simulink model "Main_2015a_ABS"  (R2015a)
settings: Solver=ode45  SolverMode=SingleTasking  StartTime=0.0  StopTime=20  MaxStep=.01  RelTol=1e-3  AbsTol=1e-6
PreLoadFcn:
  | % Load initialization data
  | 
  | sldemo_absdata;
values from neighbouring files (symbols this model uses):
  ABS_FLAG = 1    [matlab.mat]
  g = 9.8    [matlab.mat]
  I = 1.04    [matlab.mat]
  Kf = 1    [matlab.mat]
  m = 350    [matlab.mat]
  mu = [0 0.4 0.8 0.97 1 0.98 0.96 0.94 0.92 0.9 0.88 0.855 ... (21 elements, 1x21)]    [matlab.mat]
  PBmax = 1500    [matlab.mat]
  Rr = 0.356    [matlab.mat]
  slip = [0 0.05 0.1 0.15 0.2 0.25 0.3 0.35 0.4 0.45 0.5 0.55 ... (21 elements, 1x21)]    [matlab.mat]
  TB = 0.01    [matlab.mat]
  v0 = 22    [matlab.mat]
libraries: simulink_extras x4
CloseFcn:
  | % Close the plots that are still open
  | h = findobj(0, 'Name', 'ABS Speeds');
  | if ~isempty(h),
  |   close(h);
  | end;
  | 
  | h = findobj(0, 'Name', 'ABS Slip');
  | if ~isempty(h),
  |   close(h);
  | end;
  | 
  | % Clear initial conditions data to avoid cluttering the workspace
  | 
  | clear g v0 Rr Kf m PBmax TB I slip mu ctrl h;
Description:
  | Modeling an Anti-Lock Braking System (ABS)
  | 
  | *Summary*
  | 
  | This example describes a simple model for an Anti-Lock Braking System
  | (ABS). The model simulates the dynamic behavior of a vehicle
  | under hard braking conditions. The model represents a single wheel, which
  | may be replicated a number of times to create a model for a multi-wheel
  | vehicle.
  | 
  | This model uses the signal logging feature in Simulink(R). You log signals to the
  | MATLAB(R) workspace where you can analyze and view them. You can view
  | the code in sldemo_absbrakeplots.m to see how this is done.
  | 
  | In this model, the wheel speed is calculated in a separate component
  | named sldemo_wheelspeed_absbrake.
  | This component is then referenced using a Model block.  Note that both the
  | top model and the referenced model use a variable step solver, so Simulink
  | will track zero-crossings in the referenced model.
settings Model: FPTRunName=Active  CovSFcnEnable=off  ExtModeTrigMode=oneshot  ExtModeArmWhenConnect=off  ExtModeAutoUpdateStatusClock=off  Creator=The MathWorks, Inc.  LastModifiedBy=kankan
settings DataIOCC: LimitDataPoints=off  SaveOutput=off  SaveTime=off  TimeSaveName=time  SignalLoggingName=sldemo_absbrake_output
settings OptimizationCC: InlineParams=on  InlineInvariantSignals=on  ExpressionDepthLimit=2147483647  InitFltsAndDblsToZero=on  BufferReusableBoundary=off
settings DebuggingCC: SaveWithParameterizedLinksMsg=none  MultiTaskDSMMsg=warning  SigSpecEnsureSampleTimeMsg=none  IntegerOverflowMsg=none  FcnCallInpInsideContextMsg=EnableAllAsWarning  BusObjectLabelMismatch=none  StateNameClashWarn=warning  IntegerSaturationMsg=none
settings HardwareCC: TargetBitPerPointer=64  TargetLongLongMode=on  TargetIntDivRoundTo=Zero  TargetEndianess=LittleEndian  TargetWordSize=64  TargetHWDeviceType=MATLAB Host
settings ModelReferenceCC: UpdateModelReferenceTargets=IfOutOfDate

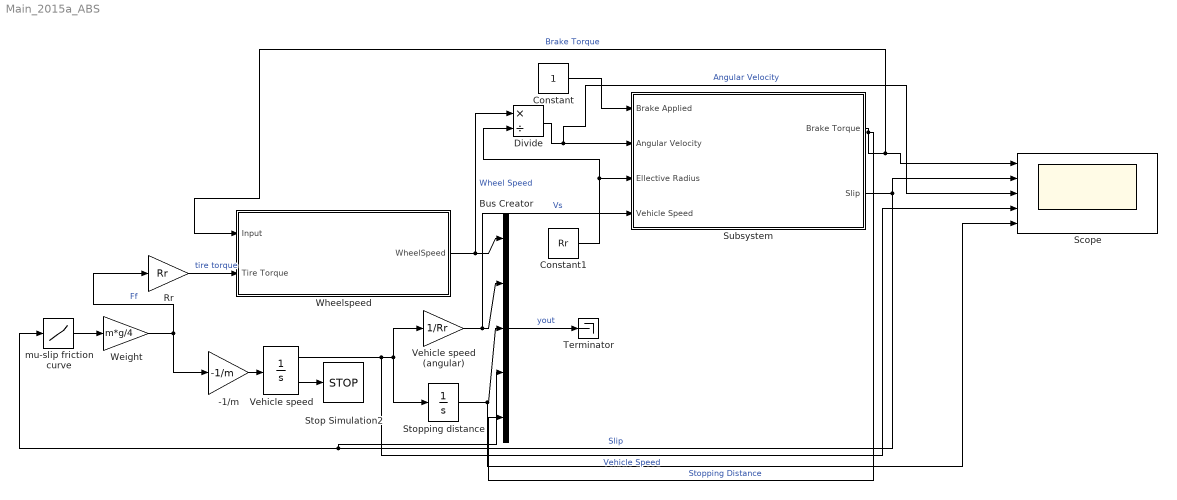
== system Main_2015a_ABS ==
  -1/m : Gain  Gain=-1/m  SaturateOnIntegerOverflow=on  OutDataTypeStr=Inherit: Same as input  ParamDataTypeStr=Inherit: Same as input
  Bus Creator : BusCreator  Inputs=5
  Constant : Constant
  Constant1 : Constant  Value=Rr
  Divide : Product  Inputs=*/
  Rr : Gain  Gain=Rr  SaturateOnIntegerOverflow=on  OutDataTypeStr=Inherit: Same as input  ParamDataTypeStr=Inherit: Same as input
  Scope : Scope  NumInputPorts=5
      settings: TimeRange=auto  MaxDataPoints=5000  SaveToWorkspace=off  SaveName=ScopeData  YMin=-2.5~-0.125~-21.69865~-2.73894~-16.73211  YMax=2.5~1.125~195.28784~24.74877~150.58895  SampleTime=-1
  Stop Simulation2 : Stop
  Stopping distance : Integrator  UpperSaturationLimit=1000  LowerSaturationLimit=0
  Subsystem : Subsystem
  Terminator : Terminator
  Vehicle speed : Integrator  InitialCondition=v0  LimitOutput=on  UpperSaturationLimit=1000  LowerSaturationLimit=0  ShowSaturationPort=on
  Vehicle speed (angular) : Gain  Gain=1/Rr  SaturateOnIntegerOverflow=on  OutDataTypeStr=Inherit: Same as input  ParamDataTypeStr=Inherit: Same as input
  Weight : Gain  Gain=m*g/4  SaturateOnIntegerOverflow=on  OutDataTypeStr=Inherit: Same as input  ParamDataTypeStr=Inherit: Same as input
  "Wheelspeed " : Subsystem
  mu-slip friction curve : Lookup_n-D  NumberOfTableDimensions=1  BreakpointsForDimension1=slip  Table=mu  SaturateOnIntegerOverflow=on  InputSameDT=on
  wires:
  Vehicle speed (angular)/1 -> Bus Creator/2, Subsystem/4(Vehicle Speed)  "Vs"
  Stopping distance/1 -> Scope/5, Bus Creator/3  "Stopping Distance"
  -1/m/1 -> Vehicle speed/1
  Vehicle speed/2 -> Stop Simulation2/1
  Vehicle speed/1 -> Scope/4, Stopping distance/1, Vehicle speed (angular)/1  "Vehicle Speed"
  mu-slip friction curve/1 -> Weight/1
  Weight/1 -> -1/m/1, Rr/1  "Ff"
  "Wheelspeed "/1(WheelSpeed) -> Divide/1, Bus Creator/1  "Wheel Speed"
  Rr/1 -> "Wheelspeed "/2(Tire Torque)  "tire torque"
  Constant/1 -> Subsystem/1(Brake Applied)
  Divide/1 -> Scope/3, Subsystem/2(Angular Velocity)  "Angular Velocity"
  Constant1/1 -> Subsystem/3(Ellective Radius), Divide/2
  Subsystem/1(Brake Torque) -> Bus Creator/5, "Wheelspeed "/1(Input), Scope/1  "Brake Torque"
  Subsystem/2(Slip) -> Scope/2, Bus Creator/4, mu-slip friction curve/1  "Slip"
  Bus Creator/1 -> Terminator/1  "yout"

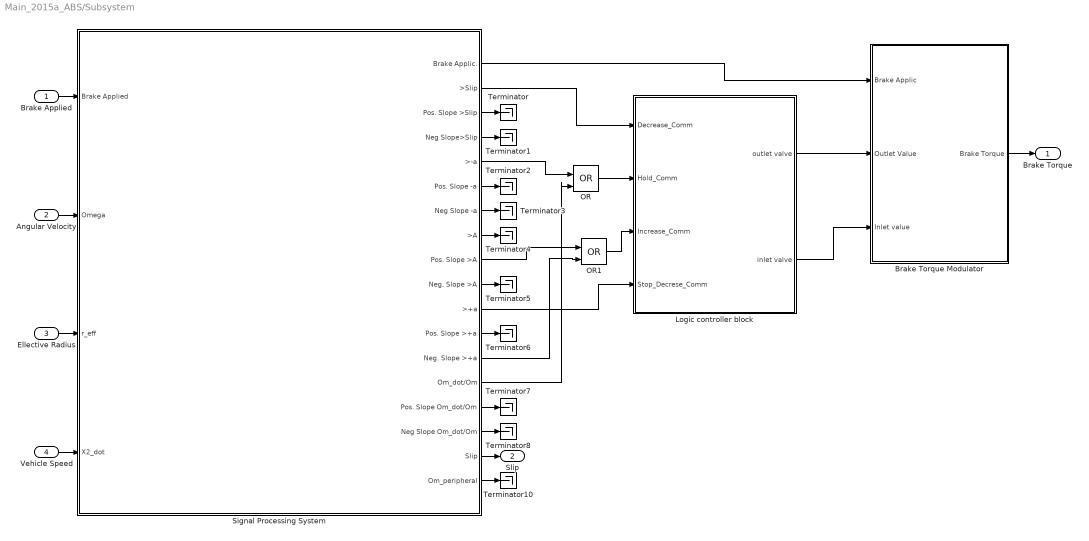
== system Main_2015a_ABS/Subsystem ==
  Brake Applied : Inport
  Angular Velocity : Inport  Port=2
  Ellective Radius : Inport  Port=3
  Vehicle Speed : Inport  Port=4
  "Brake Torque Modulator " : Subsystem
  Logic controller block : Subsystem
  OR : Logic  Operator=OR  IconShape=distinctive  AllPortsSameDT=off  OutDataTypeStr=boolean
  OR1 : Logic  Operator=OR  IconShape=distinctive  AllPortsSameDT=off  OutDataTypeStr=boolean
  Signal Processing System : Subsystem
  Terminator{,1..8,10} (10 alike) : Terminator
  Brake Torque : Outport
  Slip : Outport  Port=2
  wires:
  OR1/1 -> Logic controller block/3(Increase_Comm)
  Signal Processing System/8(>A) -> Terminator4/1
  Vehicle Speed/1 -> Signal Processing System/4(X2_dot)
  Signal Processing System/1(Brake Applic.) -> "Brake Torque Modulator "/1(Brake Applic)
  Signal Processing System/5(>-a) -> OR/1
  Brake Applied/1 -> Signal Processing System/1(Brake Applied)
  OR/1 -> Logic controller block/2(Hold_Comm)
  Signal Processing System/13(Neg. Slope >+a) -> OR1/2
  Signal Processing System/9(Pos. Slope >A) -> OR1/1
  Signal Processing System/6(Pos. Slope -a) -> Terminator2/1
  Signal Processing System/11(>+a) -> Logic controller block/4(Stop_Decrese_Comm)
  Signal Processing System/2(>Slip) -> Logic controller block/1(Decrease_Comm)
  Ellective Radius/1 -> Signal Processing System/3(r_eff)
  Logic controller block/1("outlet valve ") -> "Brake Torque Modulator "/2(Outlet Value)
  Logic controller block/2("inlet valve ") -> "Brake Torque Modulator "/3(Inlet value)
  Signal Processing System/4(Neg Slope>Slip) -> Terminator1/1
  Signal Processing System/14(Om_dot/Om) -> OR/2
  Signal Processing System/10(Neg. Slope >A) -> Terminator5/1
  Signal Processing System/12(Pos. Slope >+a) -> Terminator6/1
  Signal Processing System/15(Pos. Slope Om_dot/Om) -> Terminator7/1
  Signal Processing System/16(Neg Slope Om_dot/Om) -> Terminator8/1
  "Brake Torque Modulator "/1(Brake Torque) -> Brake Torque/1
  Signal Processing System/18("Om_peripheral ") -> Terminator10/1
  Signal Processing System/17(Slip) -> Slip/1
  Signal Processing System/7(Neg Slope -a) -> Terminator3/1
  Signal Processing System/3(Pos. Slope >Slip) -> Terminator/1
  Angular Velocity/1 -> Signal Processing System/2(Omega)

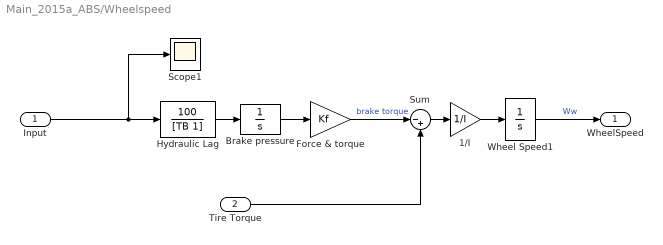
== system Main_2015a_ABS/Wheelspeed  ==
  Input : Inport  SampleTime=0
  Tire Torque : Inport  Port=2
  1/I : Gain  Gain=1/I  SaturateOnIntegerOverflow=on  OutDataTypeStr=Inherit: Same as input  ParamDataTypeStr=Inherit: Same as input
  Brake pressure : Integrator  LimitOutput=on  UpperSaturationLimit=PBmax  LowerSaturationLimit=0
  Force & torque : Gain  Gain=Kf  SaturateOnIntegerOverflow=on  OutDataTypeStr=Inherit: Same as input  ParamDataTypeStr=Inherit: Same as input
  "Hydraulic Lag " : TransferFcn  Numerator=[100]  Denominator=[TB 1]
  Scope1 : Scope
      settings: TimeRange=auto  MaxDataPoints=5000  SaveToWorkspace=off  YMin=-1.25  YMax=1.25  SampleTime=-1
  Sum : Sum  Inputs=|-+  SaturateOnIntegerOverflow=on  InputSameDT=on  OutDataTypeStr=Inherit: Same as first input
  Wheel Speed1 : Integrator  InitialCondition=v0/Rr  LimitOutput=on  UpperSaturationLimit=1000  LowerSaturationLimit=0
  WheelSpeed : Outport
  wires:
  Tire Torque/1 -> Sum/2
  Sum/1 -> 1/I/1
  Force & torque/1 -> Sum/1  "brake torque"
  "Hydraulic Lag "/1 -> Brake pressure/1
  1/I/1 -> Wheel Speed1/1
  Wheel Speed1/1 -> WheelSpeed/1  "Ww"
  Input/1 -> Scope1/1, "Hydraulic Lag "/1
  Brake pressure/1 -> Force & torque/1

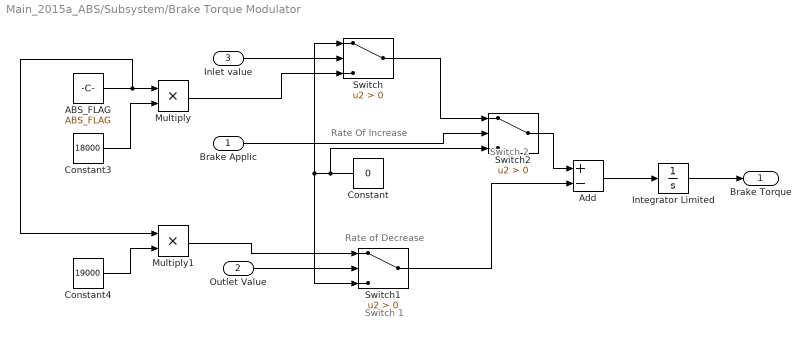
== system Main_2015a_ABS/Subsystem/Brake Torque Modulator  ==
  note: Switch 2
  note: Rate Of Increase
  note: Switch 1
  note: Rate of Decrease
  Brake Applic : Inport
  Outlet Value : Inport  Port=2
  Inlet value : Inport  Port=3
  ABS_FLAG : Constant  Value=ABS_FLAG
  Add : Sum  Inputs=+-
  Constant : Constant  Value=0
  Constant3 : Constant  Value=18000
  Constant4 : Constant  Value=19000
  Integrator Limited : Integrator  InitialCondition=1  LimitOutput=on  UpperSaturationLimit=2  LowerSaturationLimit=-2  ContinuousStateAttributes='RPM'
  Multiply : Product
  Multiply1 : Product
  Switch : Switch  Criteria=u2 > Threshold
  Switch1 : Switch  Criteria=u2 > Threshold
  Switch2 : Switch  Criteria=u2 > Threshold
  Brake Torque : Outport
  wires:
  Integrator Limited/1 -> Brake Torque/1
  Add/1 -> Integrator Limited/1
  Switch1/1 -> Add/2
  Switch2/1 -> Add/1
  Switch/1 -> Switch2/1
  Constant/1 -> Switch2/3, Switch/1, Switch1/3
  Brake Applic/1 -> Switch2/2
  Inlet value/1 -> Switch/2
  Outlet Value/1 -> Switch1/2
  ABS_FLAG/1 -> Multiply1/1, Multiply/1
  Constant3/1 -> Multiply/2
  Multiply/1 -> Switch/3
  Multiply1/1 -> Switch1/1
  Constant4/1 -> Multiply1/2

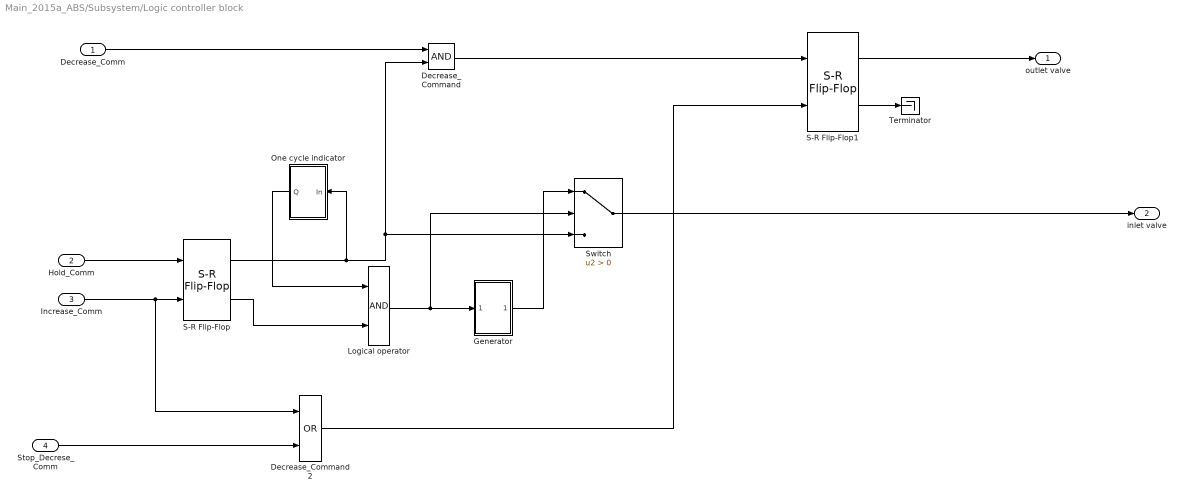
== system Main_2015a_ABS/Subsystem/Logic controller block ==
  Decrease_Comm : Inport
  Hold_Comm : Inport  Port=2
  Increase_Comm : Inport  Port=3
  Stop_Decrese_Comm : Inport  Port=4
  "Decrease_Command " : Logic  AllPortsSameDT=off  OutDataTypeStr=boolean
  Decrease_Command 2 : Logic  Operator=OR  AllPortsSameDT=off  OutDataTypeStr=boolean
  Generator : Subsystem
  "Logical operator " : Logic  AllPortsSameDT=off  OutDataTypeStr=boolean
  One cycle indicator : Subsystem
  S-R Flip-Flop : simulink_extras/Flip Flops/S-R Flip-Flop  initial_condition=0
  S-R Flip-Flop1 : simulink_extras/Flip Flops/S-R Flip-Flop  initial_condition=0
  Switch : Switch  Criteria=u2 > Threshold
  Terminator : Terminator
  "outlet valve " : Outport
  "inlet valve " : Outport  Port=2
  wires:
  Hold_Comm/1 -> S-R Flip-Flop/1
  Increase_Comm/1 -> Decrease_Command 2/1, S-R Flip-Flop/2
  Decrease_Comm/1 -> "Decrease_Command "/1
  S-R Flip-Flop/1 -> One cycle indicator/1("In "), Switch/3, "Decrease_Command "/2
  One cycle indicator/1(Q) -> "Logical operator "/1
  S-R Flip-Flop1/1 -> "outlet valve "/1
  "Decrease_Command "/1 -> S-R Flip-Flop1/1
  Switch/1 -> "inlet valve "/1
  "Logical operator "/1 -> Switch/2, Generator/1(In1)
  Stop_Decrese_Comm/1 -> Decrease_Command 2/2
  Decrease_Command 2/1 -> S-R Flip-Flop1/2
  Generator/1("out ") -> Switch/1
  S-R Flip-Flop1/2 -> Terminator/1
  S-R Flip-Flop/2 -> "Logical operator "/2

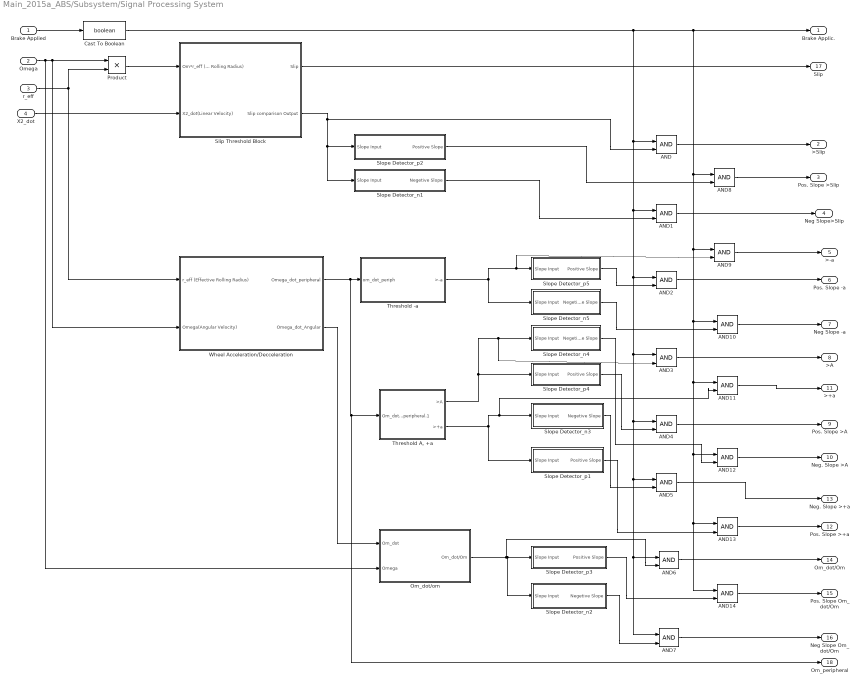
== system Main_2015a_ABS/Subsystem/Signal Processing System ==
  Brake Applied : Inport
  Omega : Inport  Port=2
  r_eff : Inport  Port=3
  X2_dot : Inport  Port=4
  AND{,1..14} (15 alike) : Logic  IconShape=distinctive  AllPortsSameDT=off  OutDataTypeStr=boolean
  Cast To Boolean : DataTypeConversion  OutDataTypeStr=boolean
  Om_dot/om : Subsystem
  Product : Product
  Slip Threshold Block : Subsystem
  Slope Detector_n1 : Subsystem
  Slope Detector_n2 : Subsystem
  Slope Detector_n3 : Subsystem
  Slope Detector_n4 : Subsystem
  Slope Detector_n5 : Subsystem
  Slope Detector_p1 : Subsystem
  Slope Detector_p2 : Subsystem
  Slope Detector_p3 : Subsystem
  Slope Detector_p4 : Subsystem
  Slope Detector_p5 : Subsystem
  Threshold -a : Subsystem
  "Threshold A, +a" : Subsystem
  Wheel Acceleration/Decceleration : Subsystem
  Brake Applic. : Outport
  >Slip : Outport  Port=2
  Pos. Slope >Slip : Outport  Port=3
  Neg Slope>Slip : Outport  Port=4
  >-a : Outport  Port=5
  Pos. Slope -a : Outport  Port=6
  Neg Slope -a : Outport  Port=7
  >A : Outport  Port=8
  Pos. Slope >A : Outport  Port=9
  Neg. Slope >A : Outport  Port=10
  >+a : Outport  Port=11
  Pos. Slope >+a : Outport  Port=12
  Neg. Slope >+a : Outport  Port=13
  Om_dot/Om : Outport  Port=14
  Pos. Slope Om_dot/Om : Outport  Port=15
  Neg Slope Om_dot/Om : Outport  Port=16
  Slip : Outport  Port=17
  "Om_peripheral " : Outport  Port=18
  wires:
  "Threshold A, +a"/2(>+a) -> AND11/2, Slope Detector_n3/1(Slope Input), Slope Detector_p1/1(Slope Input)
  Threshold -a/1(>-a) -> Slope Detector_n5/1(Slope Input), AND9/2, Slope Detector_p5/1(Slope Input)
  AND4/1 -> Pos. Slope >A/1
  AND/1 -> >Slip/1
  Product/1 -> Slip Threshold Block/1(Om*r_eff (Angular Velocity * Rolling Radius))
  Brake Applied/1 -> Cast To Boolean/1
  AND3/1 -> >A/1
  Cast To Boolean/1 -> AND/1, AND1/1, AND2/1, AND3/1, AND4/1, AND5/1, AND6/1, AND7/1, Brake Applic./1, AND8/1, AND9/1, AND10/1, AND12/1, AND13/1, AND14/1, AND11/1
  Slope Detector_n5/1(Negetive Slope) -> AND10/2
  Slip Threshold Block/2(Slip comparison Output) -> AND/2, Slope Detector_n1/1(Slope Input), Slope Detector_p2/1(Slope Input)
  r_eff/1 -> Wheel Acceleration/Decceleration/1(r_eff (Effective Rolling Radius)), Product/2
  "Threshold A, +a"/1(>A) -> AND3/2, Slope Detector_n4/1(Slope Input), Slope Detector_p4/1(Slope Input)
  Slope Detector_p2/1(Positive Slope) -> AND8/2
  AND6/1 -> Om_dot/Om/1
  Slope Detector_n2/1(Negetive Slope) -> AND7/2
  AND1/1 -> Neg Slope>Slip/1
  AND13/1 -> Pos. Slope >+a/1
  AND5/1 -> Neg. Slope >+a/1
  AND12/1 -> Neg. Slope >A/1
  AND14/1 -> Pos. Slope Om_dot/Om/1
  Om_dot/om/1(Om_dot/Om) -> AND6/2, Slope Detector_n2/1(Slope Input), Slope Detector_p3/1(Slope Input)
  Slope Detector_p5/1(Positive Slope) -> AND2/2
  AND9/1 -> >-a/1
  Omega/1 -> Om_dot/om/2(Omega), Wheel Acceleration/Decceleration/2(Omega(Angular Velocity)), Product/1
  Wheel Acceleration/Decceleration/2(Omega_dot_Angular) -> Om_dot/om/1(Om_dot)
  Slope Detector_p1/1(Positive Slope) -> AND13/2
  Slope Detector_p3/1(Positive Slope) -> AND14/2
  Slope Detector_n1/1(Negetive Slope) -> AND1/2
  AND2/1 -> Pos. Slope -a/1
  AND10/1 -> Neg Slope -a/1
  Wheel Acceleration/Decceleration/1(Omega_dot_peripheral) -> Threshold -a/1(om_dot_periph), "Om_peripheral "/1, "Threshold A, +a"/1(Om_dot_peripheral.1)
  Slip Threshold Block/1(Slip) -> Slip/1
  X2_dot/1 -> Slip Threshold Block/2(X2_dot(Linear Velocity))
  Slope Detector_p4/1(Positive Slope) -> AND4/2
  AND7/1 -> Neg Slope Om_dot/Om/1
  AND11/1 -> >+a/1
  Slope Detector_n3/1(Negetive Slope) -> AND5/2
  AND8/1 -> Pos. Slope >Slip/1
  Slope Detector_n4/1(Negetive Slope) -> AND12/2

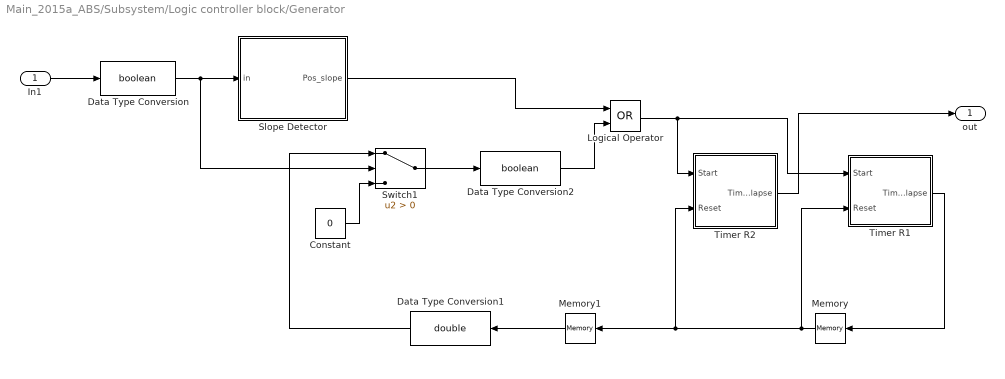
== system Main_2015a_ABS/Subsystem/Logic controller block/Generator ==
  In1 : Inport
  Constant : Constant  Value=0
  Data Type Conversion : DataTypeConversion  OutDataTypeStr=boolean
  Data Type Conversion1 : DataTypeConversion  OutDataTypeStr=double
  Data Type Conversion2 : DataTypeConversion  OutDataTypeStr=boolean
  Logical Operator : Logic  Operator=OR  AllPortsSameDT=off  OutDataTypeStr=boolean
  Memory : Memory
  Memory1 : Memory
  Slope Detector : Subsystem
  Switch1 : Switch  Criteria=u2 > Threshold
  "Timer R1 " : Subsystem
  "Timer R2 " : Subsystem
  "out " : Outport
  wires:
  Data Type Conversion1/1 -> Switch1/1
  "Timer R1 "/1(Time elapse) -> Memory/1
  In1/1 -> Data Type Conversion/1
  Constant/1 -> Switch1/3
  Data Type Conversion/1 -> Switch1/2, Slope Detector/1(in)
  Data Type Conversion2/1 -> Logical Operator/2
  Logical Operator/1 -> "Timer R1 "/1(Start), "Timer R2 "/1(Start)
  Switch1/1 -> Data Type Conversion2/1
  Memory/1 -> "Timer R2 "/2(Reset), Memory1/1, "Timer R1 "/2(Reset)
  Slope Detector/1("Pos_slope ") -> Logical Operator/1
  Memory1/1 -> Data Type Conversion1/1
  "Timer R2 "/1(Time elapse) -> "out "/1

== system Main_2015a_ABS/Subsystem/Logic controller block/One cycle indicator ==
  "In " : Inport
  Constant3 : Constant
  Switch1 : Switch  Threshold=1
  Unit Delay : UnitDelay  SampleTime=-1
  Q : Outport
  wires:
  Switch1/1 -> Q/1, Unit Delay/1
  "In "/1 -> Switch1/2
  Unit Delay/1 -> Switch1/3
  Constant3/1 -> Switch1/1

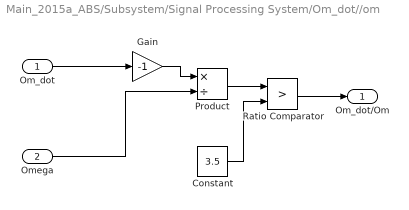
== system Main_2015a_ABS/Subsystem/Signal Processing System/Om_dot//om ==
  Om_dot : Inport
  Omega : Inport  Port=2
  Constant : Constant  Value=3.5
  Gain : Gain  Gain=-1
  Product : Product  Inputs=*/
  Ratio Comparator : RelationalOperator  Operator=>  OutDataTypeStr=boolean
  Om_dot/Om : Outport
  wires:
  Gain/1 -> Product/1
  Constant/1 -> Ratio Comparator/2
  Omega/1 -> Product/2
  Product/1 -> Ratio Comparator/1
  Om_dot/1 -> Gain/1
  Ratio Comparator/1 -> Om_dot/Om/1

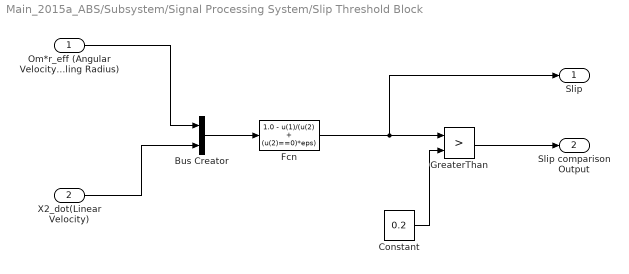
== system Main_2015a_ABS/Subsystem/Signal Processing System/Slip Threshold Block ==
  Om*r_eff (Angular Velocity * Rolling Radius) : Inport
  X2_dot(Linear Velocity) : Inport  Port=2
  Bus Creator : BusCreator  Inputs=2
  Constant : Constant  Value=0.2
  Fcn : Fcn  Expr=1.0 - u(1)/(u(2) + (u(2)==0)*eps)
  GreaterThan : RelationalOperator  Operator=>  OutDataTypeStr=boolean
  Slip : Outport
  Slip comparison Output : Outport  Port=2
  wires:
  Fcn/1 -> Slip/1, GreaterThan/1
  Constant/1 -> GreaterThan/2
  GreaterThan/1 -> Slip comparison Output/1
  Bus Creator/1 -> Fcn/1
  Om*r_eff (Angular Velocity * Rolling Radius)/1 -> Bus Creator/1
  X2_dot(Linear Velocity)/1 -> Bus Creator/2

== system Main_2015a_ABS/Subsystem/Signal Processing System/Slope Detector_n1 ==
  Slope Input : Inport
  AND : Logic  IconShape=distinctive  AllPortsSameDT=off  OutDataTypeStr=boolean
  Memory : Memory
  XOR : Logic  Operator=XOR  IconShape=distinctive  AllPortsSameDT=off  OutDataTypeStr=boolean
  Negetive Slope : Outport
  wires:
  Memory/1 -> AND/1, XOR/1
  AND/1 -> Negetive Slope/1
  Slope Input/1 -> XOR/2, Memory/1
  XOR/1 -> AND/2

== system Main_2015a_ABS/Subsystem/Signal Processing System/Slope Detector_n2 ==
  Slope Input : Inport
  AND : Logic  IconShape=distinctive  AllPortsSameDT=off  OutDataTypeStr=boolean
  Memory : Memory
  XOR : Logic  Operator=XOR  IconShape=distinctive  AllPortsSameDT=off  OutDataTypeStr=boolean
  Negetive Slope : Outport
  wires:
  Memory/1 -> AND/1, XOR/1
  AND/1 -> Negetive Slope/1
  Slope Input/1 -> XOR/2, Memory/1
  XOR/1 -> AND/2

== system Main_2015a_ABS/Subsystem/Signal Processing System/Slope Detector_n3 ==
  Slope Input : Inport
  AND : Logic  IconShape=distinctive  AllPortsSameDT=off  OutDataTypeStr=boolean
  Memory : Memory
  XOR : Logic  Operator=XOR  IconShape=distinctive  AllPortsSameDT=off  OutDataTypeStr=boolean
  Negetive Slope : Outport
  wires:
  Memory/1 -> AND/1, XOR/1
  AND/1 -> Negetive Slope/1
  Slope Input/1 -> XOR/2, Memory/1
  XOR/1 -> AND/2

== system Main_2015a_ABS/Subsystem/Signal Processing System/Slope Detector_n4 ==
  Slope Input : Inport
  AND : Logic  IconShape=distinctive  AllPortsSameDT=off  OutDataTypeStr=boolean
  Memory : Memory
  XOR : Logic  Operator=XOR  IconShape=distinctive  AllPortsSameDT=off  OutDataTypeStr=boolean
  Negetive Slope : Outport
  wires:
  Memory/1 -> AND/1, XOR/1
  AND/1 -> Negetive Slope/1
  Slope Input/1 -> XOR/2, Memory/1
  XOR/1 -> AND/2

== system Main_2015a_ABS/Subsystem/Signal Processing System/Slope Detector_n5 ==
  Slope Input : Inport
  AND : Logic  IconShape=distinctive  AllPortsSameDT=off  OutDataTypeStr=boolean
  Memory : Memory
  XOR : Logic  Operator=XOR  IconShape=distinctive  AllPortsSameDT=off  OutDataTypeStr=boolean
  Negetive Slope : Outport
  wires:
  Memory/1 -> AND/1, XOR/1
  AND/1 -> Negetive Slope/1
  Slope Input/1 -> XOR/2, Memory/1
  XOR/1 -> AND/2

== system Main_2015a_ABS/Subsystem/Signal Processing System/Slope Detector_p1 ==
  Slope Input : Inport
  AND : Logic  IconShape=distinctive  AllPortsSameDT=off  OutDataTypeStr=boolean
  Memory : Memory
  XOR : Logic  Operator=XOR  IconShape=distinctive  AllPortsSameDT=off  OutDataTypeStr=boolean
  Positive Slope : Outport
  wires:
  Memory/1 -> XOR/1
  AND/1 -> Positive Slope/1
  Slope Input/1 -> AND/1, XOR/2, Memory/1
  XOR/1 -> AND/2

== system Main_2015a_ABS/Subsystem/Signal Processing System/Slope Detector_p2 ==
  Slope Input : Inport
  AND : Logic  IconShape=distinctive  AllPortsSameDT=off  OutDataTypeStr=boolean
  Memory : Memory
  XOR : Logic  Operator=XOR  IconShape=distinctive  AllPortsSameDT=off  OutDataTypeStr=boolean
  Positive Slope : Outport
  wires:
  Memory/1 -> XOR/1
  AND/1 -> Positive Slope/1
  Slope Input/1 -> AND/1, XOR/2, Memory/1
  XOR/1 -> AND/2

== system Main_2015a_ABS/Subsystem/Signal Processing System/Slope Detector_p3 ==
  Slope Input : Inport
  AND : Logic  IconShape=distinctive  AllPortsSameDT=off  OutDataTypeStr=boolean
  Memory : Memory
  XOR : Logic  Operator=XOR  IconShape=distinctive  AllPortsSameDT=off  OutDataTypeStr=boolean
  Positive Slope : Outport
  wires:
  Memory/1 -> XOR/1
  AND/1 -> Positive Slope/1
  Slope Input/1 -> AND/1, XOR/2, Memory/1
  XOR/1 -> AND/2

== system Main_2015a_ABS/Subsystem/Signal Processing System/Slope Detector_p4 ==
  Slope Input : Inport
  AND : Logic  IconShape=distinctive  AllPortsSameDT=off  OutDataTypeStr=boolean
  Memory : Memory
  XOR : Logic  Operator=XOR  IconShape=distinctive  AllPortsSameDT=off  OutDataTypeStr=boolean
  Positive Slope : Outport
  wires:
  Memory/1 -> XOR/1
  AND/1 -> Positive Slope/1
  Slope Input/1 -> AND/1, XOR/2, Memory/1
  XOR/1 -> AND/2

== system Main_2015a_ABS/Subsystem/Signal Processing System/Slope Detector_p5 ==
  Slope Input : Inport
  AND : Logic  IconShape=distinctive  AllPortsSameDT=off  OutDataTypeStr=boolean
  Memory : Memory
  XOR : Logic  Operator=XOR  IconShape=distinctive  AllPortsSameDT=off  OutDataTypeStr=boolean
  Positive Slope : Outport
  wires:
  Memory/1 -> XOR/1
  AND/1 -> Positive Slope/1
  Slope Input/1 -> AND/1, XOR/2, Memory/1
  XOR/1 -> AND/2

== system Main_2015a_ABS/Subsystem/Signal Processing System/Threshold -a ==
  om_dot_periph : Inport
  -a comparator : RelationalOperator  OutDataTypeStr=boolean
  "-a negetive acc " : Constant  Value=-60
  Gain : Gain  Gain=-1
  >-a : Outport
  wires:
  "-a negetive acc "/1 -> -a comparator/2
  om_dot_periph/1 -> Gain/1
  Gain/1 -> -a comparator/1
  -a comparator/1 -> >-a/1

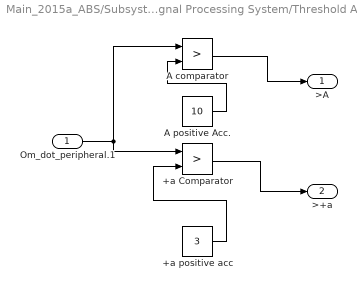
== system Main_2015a_ABS/Subsystem/Signal Processing System/Threshold A, +a ==
  Om_dot_peripheral.1 : Inport
  +a Comparator : RelationalOperator  Operator=>  OutDataTypeStr=boolean
  +a positive acc : Constant  Value=3
  A comparator : RelationalOperator  Operator=>  OutDataTypeStr=boolean
  A positive Acc. : Constant  Value=10
  >A : Outport
  >+a : Outport  Port=2
  wires:
  Om_dot_peripheral.1/1 -> +a Comparator/1, A comparator/1
  A comparator/1 -> >A/1
  A positive Acc./1 -> A comparator/2
  +a positive acc/1 -> +a Comparator/2
  +a Comparator/1 -> >+a/1

== system Main_2015a_ABS/Subsystem/Signal Processing System/Wheel Acceleration//Decceleration ==
  r_eff (Effective Rolling Radius) : Inport
  Omega(Angular Velocity) : Inport  Port=2
  Derivative : Derivative
  Low ppass : TransferFcn  Numerator=[1.15]  Denominator=[0.0105 1]
  Product : Product
  Omega_dot_peripheral : Outport
  Omega_dot_Angular : Outport  Port=2
  wires:
  Omega(Angular Velocity)/1 -> Derivative/1
  Low ppass/1 -> Omega_dot_Angular/1, Product/2
  Product/1 -> Omega_dot_peripheral/1
  Derivative/1 -> Low ppass/1
  r_eff (Effective Rolling Radius)/1 -> Product/1

== system Main_2015a_ABS/Subsystem/Logic controller block/Generator/Slope Detector ==
  in : Inport
  Logical Operator : Logic  AllPortsSameDT=off  OutDataTypeStr=boolean
  Logical Operator1 : Logic  Operator=XOR  AllPortsSameDT=off  OutDataTypeStr=boolean
  Memory1 : Memory
  "Pos_slope " : Outport
  wires:
  Logical Operator/1 -> "Pos_slope "/1
  in/1 -> Logical Operator1/2, Logical Operator/1, Memory1/1
  Memory1/1 -> Logical Operator1/1
  Logical Operator1/1 -> Logical Operator/2

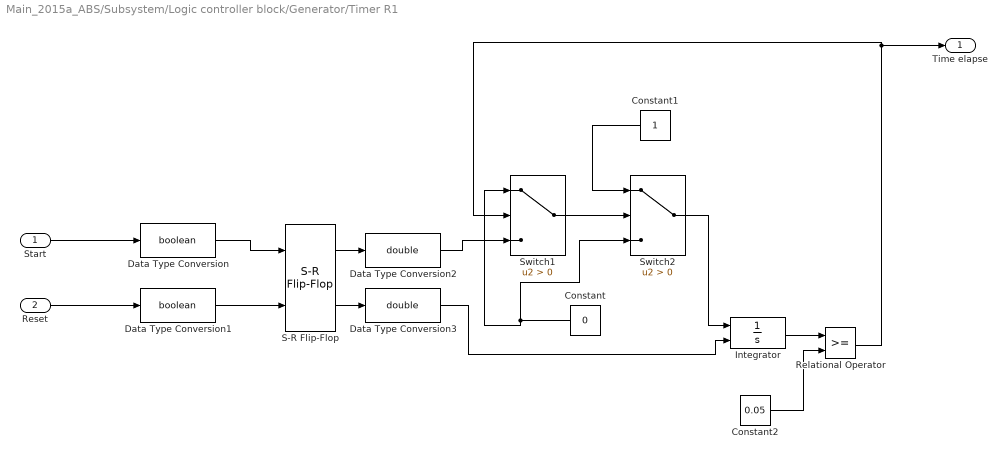
== system Main_2015a_ABS/Subsystem/Logic controller block/Generator/Timer R1  ==
  Start : Inport
  Reset : Inport  Port=2
  Constant : Constant  Value=0
  Constant1 : Constant
  Constant2 : Constant  Value=0.05
  Data Type Conversion : DataTypeConversion  OutDataTypeStr=boolean
  Data Type Conversion1 : DataTypeConversion  OutDataTypeStr=boolean
  Data Type Conversion2 : DataTypeConversion  OutDataTypeStr=double
  Data Type Conversion3 : DataTypeConversion  OutDataTypeStr=double
  Integrator : Integrator  ExternalReset=level
  Relational Operator : RelationalOperator  OutDataTypeStr=boolean
  S-R Flip-Flop : simulink_extras/Flip Flops/S-R Flip-Flop  initial_condition=0
  Switch1 : Switch  Criteria=u2 > Threshold
  Switch2 : Switch  Criteria=u2 > Threshold
  Time elapse : Outport
  wires:
  Data Type Conversion/1 -> S-R Flip-Flop/1
  Start/1 -> Data Type Conversion/1
  Reset/1 -> Data Type Conversion1/1
  Constant1/1 -> Switch2/1
  Switch1/1 -> Switch2/2
  Switch2/1 -> Integrator/1
  Relational Operator/1 -> Time elapse/1, Switch1/2
  Constant/1 -> Switch1/1, Switch2/3
  Integrator/1 -> Relational Operator/1
  Data Type Conversion2/1 -> Switch1/3
  Constant2/1 -> Relational Operator/2
  Data Type Conversion3/1 -> Integrator/2
  Data Type Conversion1/1 -> S-R Flip-Flop/2
  S-R Flip-Flop/1 -> Data Type Conversion2/1
  S-R Flip-Flop/2 -> Data Type Conversion3/1

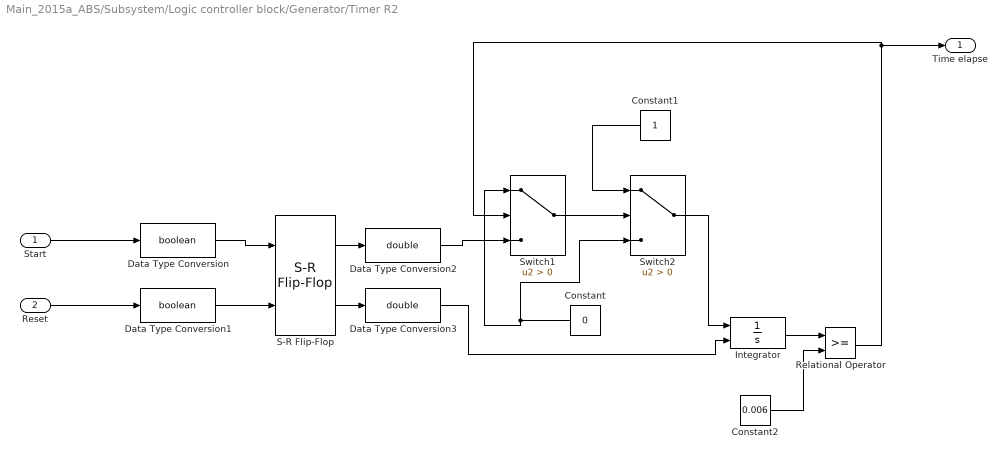
== system Main_2015a_ABS/Subsystem/Logic controller block/Generator/Timer R2  ==
  Start : Inport
  Reset : Inport  Port=2
  Constant : Constant  Value=0
  Constant1 : Constant
  Constant2 : Constant  Value=0.006
  Data Type Conversion : DataTypeConversion  OutDataTypeStr=boolean
  Data Type Conversion1 : DataTypeConversion  OutDataTypeStr=boolean
  Data Type Conversion2 : DataTypeConversion  OutDataTypeStr=double
  Data Type Conversion3 : DataTypeConversion  OutDataTypeStr=double
  Integrator : Integrator  ExternalReset=level
  Relational Operator : RelationalOperator  OutDataTypeStr=boolean
  S-R Flip-Flop : simulink_extras/Flip Flops/S-R Flip-Flop  initial_condition=0
  Switch1 : Switch  Criteria=u2 > Threshold
  Switch2 : Switch  Criteria=u2 > Threshold
  Time elapse : Outport
  wires:
  Data Type Conversion3/1 -> Integrator/2
  Constant2/1 -> Relational Operator/2
  Data Type Conversion2/1 -> Switch1/3
  Integrator/1 -> Relational Operator/1
  Constant/1 -> Switch2/3, Switch1/1
  Relational Operator/1 -> Switch1/2, Time elapse/1
  Switch2/1 -> Integrator/1
  Switch1/1 -> Switch2/2
  Constant1/1 -> Switch2/1
  Reset/1 -> Data Type Conversion1/1
  Start/1 -> Data Type Conversion/1
  Data Type Conversion/1 -> S-R Flip-Flop/1
  S-R Flip-Flop/1 -> Data Type Conversion2/1
  Data Type Conversion1/1 -> S-R Flip-Flop/2
  S-R Flip-Flop/2 -> Data Type Conversion3/1
